simulink library "sdf"  (Simulink 8.1)
settings: Solver=ode1  StartTime=0.0  StopTime=Inf  FixedStep=0.001  RelTol=1e-3
PostLoadFcn:
  | , if any(exist('dsrtsu_mdlpostloadfcn', 'file') == [2, 3, 6]), try dsrtsu_mdlpostloadfcn('Execute', bdroot); catch fprintf('Error in PostLoadFcn (dsrtsu_mdlpostloadfcn) for model "%s":\n %s\n', bdroot, lasterr); end, end,
settings Model: DSRTSU_INTERNAL_RTI_VER=450  DSRTSU_INTERNAL_RTI_TYPE=rti1401  RTICANMMDATA=struct('GeneralSetupData',struct('modelroot','D:\PROJECTS\HAITEC\TAIWAN_HAITEC_SVN\branches\Model_with_Distance_trigger\AdasDragon\software\sw_development\arch\app\per','generalsettings',struct('filesettings',struct('destfolder',struct('Name','RTICANMM_FILES','Check',1),'buildfolder',struct('Name','.','Check',1),'AbsDestfolder',struct('Name','D:\PROJECTS\HAITEC\TAIWAN_HAITEC_SVN\branches\Model_with_Distance_trigger\AdasDragon\software\sw_development\arch\app\per\RTICANMM_FILES'),'AbsBuildfolder',struct('Name','D:\PROJECTS\HAITEC\TAIWAN_HAITEC_SVN\branches\Model_with_Distance_trigger\AdasDragon\software\sw_development\arch\app\per'))),'options',struct('addpaths',1,'rmpaths',1,'addtrcexclusion',logical(1),'cannavigator',struct('checkmonitoring',0),'show_usrtrc',0,'use_usrtrc',0),'advanced',struct('options',[1 1 1 1 1 1 1 1 1 1 1 1 1 1 1 1 1 1 1 1 1 1 1 1 1 1 1 1 1 1 1 1 1 1 1 1 1 1 1 1 1 1 1 1 1 1 1 1 1 1 1 1 1 1 1 1 1 1 1 1 1 1 1 1 1 1 1 1 1 1 1 1 1 1 1 1 1 1 1 1 1 1 1 1 1 1 1 1 1 1 1 1 1 1 1 1 1 1 1 1]),'MPSetup',{{}},'modelname','sdf','block','sdf'))  DSRTSU_INTERNAL_RTIFPGA=40  Creator=AT015086  LastModifiedBy=tescamilla

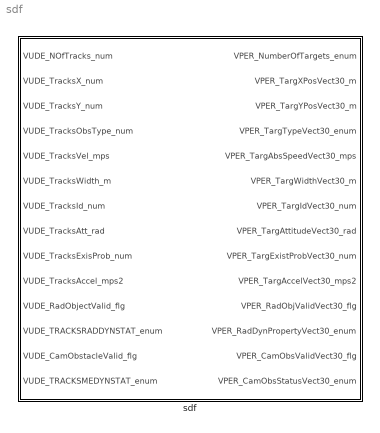
== system sdf ==
  sdf : Subsystem

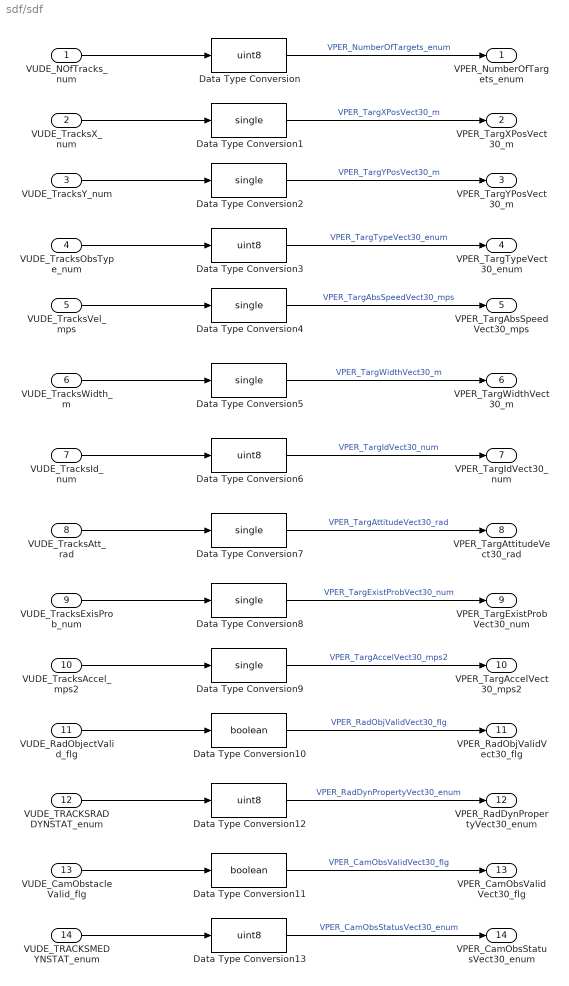
== system sdf/sdf ==
  VUDE_NOfTracks_num : Inport
  VUDE_TracksX_num : Inport  Port=2
  VUDE_TracksY_num : Inport  Port=3
  VUDE_TracksObsType_num : Inport  Port=4
  VUDE_TracksVel_mps : Inport  Port=5
  VUDE_TracksWidth_m : Inport  Port=6
  VUDE_TracksId_num : Inport  Port=7
  VUDE_TracksAtt_rad : Inport  Port=8
  VUDE_TracksExisProb_num : Inport  Port=9
  VUDE_TracksAccel_mps2 : Inport  Port=10
  VUDE_RadObjectValid_flg : Inport  Port=11
  VUDE_TRACKSRADDYNSTAT_enum : Inport  Port=12
  VUDE_CamObstacleValid_flg : Inport  Port=13
  VUDE_TRACKSMEDYNSTAT_enum : Inport  Port=14
  Data Type Conversion{,3,6,12..13} (5 alike) : DataTypeConversion  OutDataTypeStr=uint8
  Data Type Conversion{1..2,4..5,7..9} (7 alike) : DataTypeConversion  OutDataTypeStr=single
  Data Type Conversion10 : DataTypeConversion  OutDataTypeStr=boolean
  Data Type Conversion11 : DataTypeConversion  OutDataTypeStr=boolean
  VPER_NumberOfTargets_enum : Outport
  VPER_TargXPosVect30_m : Outport  Port=2
  VPER_TargYPosVect30_m : Outport  Port=3
  VPER_TargTypeVect30_enum : Outport  Port=4
  VPER_TargAbsSpeedVect30_mps : Outport  Port=5
  VPER_TargWidthVect30_m : Outport  Port=6
  VPER_TargIdVect30_num : Outport  Port=7
  VPER_TargAttitudeVect30_rad : Outport  Port=8
  VPER_TargExistProbVect30_num : Outport  Port=9
  VPER_TargAccelVect30_mps2 : Outport  Port=10
  VPER_RadObjValidVect30_flg : Outport  Port=11
  VPER_RadDynPropertyVect30_enum : Outport  Port=12
  VPER_CamObsValidVect30_flg : Outport  Port=13
  VPER_CamObsStatusVect30_enum : Outport  Port=14
  wires:
  VUDE_NOfTracks_num/1 -> Data Type Conversion/1
  VUDE_TracksY_num/1 -> Data Type Conversion2/1
  Data Type Conversion3/1 -> VPER_TargTypeVect30_enum/1  "VPER_TargTypeVect30_enum"
  VUDE_TracksVel_mps/1 -> Data Type Conversion4/1
  Data Type Conversion5/1 -> VPER_TargWidthVect30_m/1  "VPER_TargWidthVect30_m"
  Data Type Conversion2/1 -> VPER_TargYPosVect30_m/1  "VPER_TargYPosVect30_m"
  VUDE_TracksObsType_num/1 -> Data Type Conversion3/1
  Data Type Conversion/1 -> VPER_NumberOfTargets_enum/1  "VPER_NumberOfTargets_enum"
  VUDE_TracksWidth_m/1 -> Data Type Conversion5/1
  VUDE_TracksX_num/1 -> Data Type Conversion1/1
  Data Type Conversion1/1 -> VPER_TargXPosVect30_m/1  "VPER_TargXPosVect30_m"
  Data Type Conversion4/1 -> VPER_TargAbsSpeedVect30_mps/1  "VPER_TargAbsSpeedVect30_mps"
  VUDE_TracksId_num/1 -> Data Type Conversion6/1
  VUDE_TracksAtt_rad/1 -> Data Type Conversion7/1
  VUDE_TracksExisProb_num/1 -> Data Type Conversion8/1
  Data Type Conversion6/1 -> VPER_TargIdVect30_num/1  "VPER_TargIdVect30_num"
  Data Type Conversion7/1 -> VPER_TargAttitudeVect30_rad/1  "VPER_TargAttitudeVect30_rad"
  Data Type Conversion8/1 -> VPER_TargExistProbVect30_num/1  "VPER_TargExistProbVect30_num"
  VUDE_TracksAccel_mps2/1 -> Data Type Conversion9/1
  Data Type Conversion9/1 -> VPER_TargAccelVect30_mps2/1  "VPER_TargAccelVect30_mps2"
  VUDE_RadObjectValid_flg/1 -> Data Type Conversion10/1
  Data Type Conversion10/1 -> VPER_RadObjValidVect30_flg/1  "VPER_RadObjValidVect30_flg"
  VUDE_CamObstacleValid_flg/1 -> Data Type Conversion11/1
  Data Type Conversion11/1 -> VPER_CamObsValidVect30_flg/1  "VPER_CamObsValidVect30_flg"
  VUDE_TRACKSRADDYNSTAT_enum/1 -> Data Type Conversion12/1
  Data Type Conversion12/1 -> VPER_RadDynPropertyVect30_enum/1  "VPER_RadDynPropertyVect30_enum"
  VUDE_TRACKSMEDYNSTAT_enum/1 -> Data Type Conversion13/1
  Data Type Conversion13/1 -> VPER_CamObsStatusVect30_enum/1  "VPER_CamObsStatusVect30_enum"
